simulink model "Model_3b_NH3_Flexible_clean"  (R2019a)
settings: Solver=FixedStepAuto  StartTime=0.0  StopTime=8760  FixedStep=1  RelTol=1e-3
libraries: simulink x8
settings Model: Creator=senja  LastModifiedBy=senja

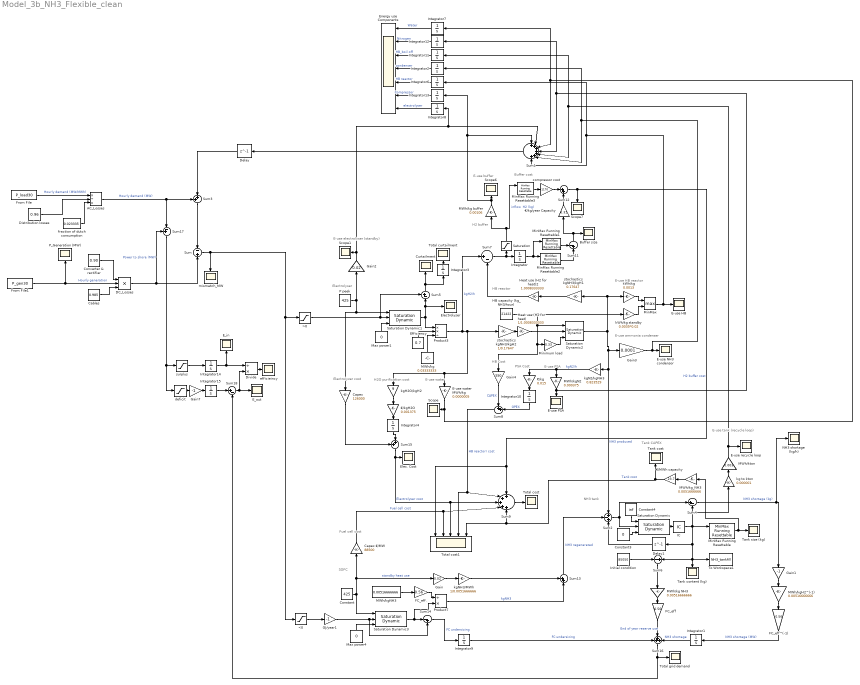
== system Model_3b_NH3_Flexible_clean ==
  note: PSA Cost
  note: H2O purification cost
  note: E-use buffer
  note: Buffer cost
  note: E-use HB reactor
  note: E-use PSA
  note: HB Cost
  note: Tank CAPEX
  note: E-use tank (recycle loop)
  note: E-use ammonia condenser
  note: NH3 tank
  note: HB reactor
  note: E-use electrolyser (standby)
  note: E-use water
  note: Fuel cell cost
  note: SOFC
  note: Electrolyser
  note: Electrolyzer cost
  note: H2 buffer
  " Heat use (H2 for heat)" : Gain  Gain=1/1.0008333333
  " Heat use (H2 for heat)2" : Gain  Gain=1.0008333333
  <0 : Saturate  UpperLimit=inf  LowerLimit=0
  >0 : Saturate  UpperLimit=inf  LowerLimit=0
  AC_Losses : Product  Inputs=*/*
  Buffer size : Scope
  Cables : Constant  Value=0.985
  Capex : Gain  Gain=126000
  Capex €/MW : Gain  Gain=88500
  Constant : Constant  Value=425
  Constant3 : Constant  Value=0
  Constant4 : Constant  Value=inf
  Converter & rectifier : Constant  Value=0.90
  Curtailment : Scope
  DC_Losses : Product  Inputs=3
  Delay : Delay  DelayLength=1  InitialCondition=0
  Delay1 : Delay  DelayLength=1
  Distribution losses : Constant  Value=0.96
  Divide : Product  Inputs=/*
  E-use HB : Scope
  E-use NH3 condensor : Scope
  E-use PSA : Scope
  E-use recycle loop : Scope
  E-use water MWh/kg : Gain  Gain=0.0000005
  E_in : Scope
  E_out : Scope
  Efficiency : Constant  Value=0.7
  Elec. Cost : Scope
  Electrolyser : Scope
  Energy use Components : Scope  NumInputPorts=7
  "FC_eff " : Gain  Gain=0.56
  FC_eff. : Gain  Gain=0.56
  FC_eff^(-1) : Gain  Gain=0.56
  From File : FromFile  FileName=P_load30  SampleTime=0
  From File1 : FromFile  FileName=P_gen30  SampleTime=0
  GJ/year1 : Gain  Gain=-1
  Gain : Gain  Gain=0.02
  Gain1 : Gain  Gain=-1
  Gain2 : Gain  Gain=0.02
  Gain3 : Gain  Gain=0.0001
  Gain4 : Gain  Gain=550
  Gain7 : Gain  Gain=-1
  HB capacity (kg_NH3/hour) : Constant  Value=21422
  IC : InitialCondition  Value=85050
  Initial condition : Constant  Value=85050
  Integrator{,1..4,6..15} (15 alike) : Integrator
  MWh/kg : Constant  Value=0.03333333
  MWh/kg buffer : Gain  Gain=0.00106
  MWh/kg NH3 : Gain  Gain=0.00516666666
  MWh/kgH2^(-1) : Gain  Gain=0.00516666666
  MWh/kgN2 : Gain  Gain=0.000375
  MWh/kgNH3 : Constant  Value=0.00516666666
  MWh/kg_NH3 : Gain  Gain=0.0051666666
  MWh/kton : Gain  Gain=0.003
  Max power1 : Constant  Value=0
  Max power4 : Constant  Value=0
  MinMax : MinMax  Function=max  Inputs=2
  MinMax Running Resettable : simulink/Math Operations/MinMax Running Resettable  Function=max  vinit=0.0
  MinMax Running Resettable1 : simulink/Math Operations/MinMax Running Resettable  Function=min  vinit=0.0
  MinMax Running Resettable2 : simulink/Math Operations/MinMax Running Resettable  Function=max  vinit=0.0
  MinMax Running Resettable3 : simulink/Math Operations/MinMax Running Resettable  Function=max  vinit=0.0
  Minimum load : Gain  Gain=0.33
  NH3 shortage (kg/h) : Scope
  P peek : Constant  Value=425
  P_Generation (MW) : Scope
  Product3 : Product  Inputs=**/
  Product7 : Product  Inputs=/*
  Saturation : Saturate  UpperLimit=inf  LowerLimit=0
  Saturation Dynamic{,1..3} (4 alike) : simulink/Discontinuities/Saturation Dynamic  OutMin=[]  OutMax=[]  OutDataTypeStr=Inherit: Same as second input  OutDataType=fixdt(1, 16)  OutScaling=2^-10  DoSatur=off
  Scope{,1,6..7} (4 alike) : Scope
  Sum : Sum  Inputs=-|+
  Sum1 : Sum  Inputs=+++++++
  Sum11 : Sum  Inputs=-+|
  Sum12 : Sum  Inputs=|++
  Sum{3,8,13,15} (4 alike) : Sum  Inputs=++|
  Sum14 : Sum  Inputs=|-+
  Sum16 : Sum  Inputs=+++
  Sum17 : Sum  Inputs=+-|
  Sum18 : Sum  Inputs=|+-
  Sum2 : Sum  Inputs=+-+
  Sum4 : Sum  Inputs=|+-
  Sum5 : Sum  Inputs=+-|
  Sum6 : Sum  Inputs=-|+
  Sum7 : Sum  Inputs=|+-
  Sum9 : Sum  Inputs=+++++
  Tank content (kg) : Scope
  Tank cost : Scope
  Tank size (kg) : Scope
  To Workspace1 : ToWorkspace  VariableName=NH3_tankfill  SampleTime=-1
  Total cost : Scope
  Total cost1 : Scope  NumInputPorts=5
  Total curtailment : Scope
  Total grid demand : Scope
  compressor cost : Gain  Gain=1170
  deficit : Saturate  UpperLimit=0  LowerLimit=-inf
  efficieincy : Scope
  fraction of dutch consumption : Constant  Value=0.023335
  kWh/kg : Gain  Gain=0.0013
  kWh/kg standby : Gain  Gain=0.0035*0.02
  kg to kton : Gain  Gain=0.000001
  kgH2O/kgH2 : Gain  Gain=9
  kgN2/kgNH3 : Gain  Gain=0.823529
  kgNH3/MWh : Gain  Gain=1/0.0051666666
  mismatch_MW : Scope
  stochastics kgNH3/kgH1 : Gain  Gain=0.17647
  stochastics kgNH3/kgH2 : Gain  Gain=1/0.17647
  surplus : Saturate  UpperLimit=inf  LowerLimit=0
  €/MWh capacity : Gain  Gain=23.7
  €/kg : Gain  Gain=0.015
  €/kg/year Capacity : Gain  Gain=0.31
  €/kgH2O : Gain  Gain=0.001375
  wires:
  From File/1 -> AC_Losses/1  "Hourly demand (MW/MWh)"
  Efficiency/1 -> Product3/2
  fraction of dutch consumption/1 -> AC_Losses/3
  Distribution losses/1 -> AC_Losses/2
  Cables/1 -> DC_Losses/3
  Converter & rectifier/1 -> DC_Losses/1
  DC_Losses/1 -> Sum/2, Sum17/1  "Power to shore (MW)"
  >0/1 -> Sum5/1, Saturation Dynamic1/2
  <0/1 -> GJ/year1/1
  AC_Losses/1 -> Sum3/1, Sum17/2  "Hourly demand (MW)"
  From File1/1 -> P_Generation (MW)/1, DC_Losses/2  "Hourly generation"
  Max power1/1 -> Saturation Dynamic1/3
  Saturation Dynamic1/1 -> Electrolyser/1, Sum5/2, Product3/1
  Capex/1 -> Sum15/1
  Sum15/1 -> Elec. Cost/1, Total cost1/3, Sum9/3  "Electrolyser cost"
  €/kgH2O/1 -> Integrator4/1
  P peek/1 -> Saturation Dynamic1/1, Capex/1, Gain2/1
  GJ/year1/1 -> Saturation Dynamic3/2, Sum14/2
  Product3/1 -> stochastics kgNH3/kgH2/1, E-use water MWh/kg/1, kgH2O/kgH2/1, Sum7/1  "kgH2/h"
  Sum/1 -> <0/1, >0/1, mismatch_MW/1
  Sum9/1 -> Total cost/1
  Constant/1 -> Saturation Dynamic3/1, Capex €/MW/1, Gain/1  "standby heat use"
  Max power4/1 -> Saturation Dynamic3/3
  Saturation Dynamic3/1 -> Sum14/1, Product7/2
  MWh/kgNH3/1 -> FC_eff./1
  Integrator3/1 -> Total curtailment/1
  kgH2O/kgH2/1 -> €/kgH2O/1
  Integrator4/1 -> Sum15/2
  MWh/kg/1 -> Product3/3
  Capex €/MW/1 -> Total cost1/2, Sum9/4  "Fuel cell cost"
  FC_eff./1 -> Product7/1
  Sum5/1 -> Curtailment/1, Integrator3/1
  E-use water MWh/kg/1 -> Sum1/3, Integrator7/1, Scope/1
  Gain2/1 -> Integrator8/1, Sum1/2, Scope1/1
  Sum3/1 -> Sum/1
  Sum1/1 -> Delay/1
  Delay/1 -> Sum3/2
  Integrator2/1 -> Energy use Components/4  "condenser"
  Integrator6/1 -> Energy use Components/5  "HB reactor"
  Integrator7/1 -> Energy use Components/1  "Water"
  Integrator8/1 -> Energy use Components/7  "electrolyser"
  Product7/1 -> Sum13/2  "kgNH3"
  Sum7/1 -> Integrator/1, Saturation/1
  Integrator/1 -> MinMax Running Resettable1/1, MinMax Running Resettable2/1
  stochastics kgNH3/kgH2/1 -> " Heat use (H2 for heat)"/1
  HB capacity (kg_NH3/hour)/1 -> Saturation Dynamic2/1, Gain4/1, Minimum load/1, kWh/kg standby/1
  Sum2/1 -> Sum4/1, Saturation Dynamic/2
  Delay1/1 -> Sum2/3
  Constant3/1 -> Saturation Dynamic/3
  Sum4/1 -> NH3 shortage (kg/h)/1, Gain1/1  "NH3 shortage (kg)"
  MWh/kgH2^(-1)/1 -> FC_eff^(-1)/1
  FC_eff^(-1)/1 -> Integrator1/1  "NH3 shortage (MW)"
  Saturation Dynamic/1 -> IC/1
  IC/1 -> Sum4/2, kg to kton/1, Tank content (kg)/1, Sum6/2, To Workspace1/1, Delay1/1, MinMax Running Resettable/1
  Initial condition/1 -> Sum6/1
  Sum14/1 -> Integrator9/1  "FC undersizing"
  MWh/kg NH3/1 -> "FC_eff "/1
  "FC_eff "/1 -> Sum16/2  "End of year reserve use"
  Sum6/1 -> MWh/kg NH3/1
  Gain1/1 -> MWh/kgH2^(-1)/1
  Integrator9/1 -> Sum16/1  "FC undersizing"
  Constant4/1 -> Saturation Dynamic/1
  MinMax Running Resettable/1 -> Tank size (kg)/1, MWh/kg_NH3/1
  Gain3/1 -> Sum1/6, Integrator2/1, E-use NH3 condensor/1
  MWh/kton/1 -> Sum1/5, Integrator11/1, E-use recycle loop/1
  kg to kton/1 -> MWh/kton/1
  MWh/kg_NH3/1 -> €/MWh capacity/1
  €/MWh capacity/1 -> Total cost1/5, Sum9/5, Tank cost/1  "Tank cost"
  Gain4/1 -> Sum8/1  "CAPEX"
  kgN2/kgNH3/1 -> MWh/kgN2/1, €/kg/1  "kgN2/h"
  €/kg/1 -> Integrator10/1
  Sum8/1 -> Total cost1/4, Sum9/2  "HB reactorr cost"
  Integrator10/1 -> Sum8/2  "OPEX"
  kWh/kg/1 -> MinMax/1
  Integrator12/1 -> Energy use Components/2  "Nitrogen"
  Integrator11/1 -> Energy use Components/3  "HB_boil off"
  MWh/kgN2/1 -> Sum1/4, Integrator12/1, E-use PSA/1
  MinMax Running Resettable1/1 -> Sum11/1
  MinMax Running Resettable2/1 -> Sum11/2
  Sum11/1 -> Buffer size/1, €/kg/year Capacity/1
  €/kg/year Capacity/1 -> Sum12/2
  MWh/kg buffer/1 -> Sum1/1, Integrator13/1, Scope6/1
  Saturation/1 -> MinMax Running Resettable3/1, MWh/kg buffer/1  "inflow  H2 (kg)"
  MinMax Running Resettable3/1 -> compressor cost/1
  compressor cost/1 -> Sum12/1
  Sum12/1 -> Scope7/1, Total cost1/1, Sum9/1  "H2 buffer cost"
  Integrator13/1 -> Energy use Components/6  "Compressor"
  Sum13/1 -> Sum2/2  "NH3 regenerated"
  Gain/1 -> kgNH3/MWh/1
  kgNH3/MWh/1 -> Sum13/1
  kWh/kg standby/1 -> MinMax/2
  MinMax/1 -> Sum1/7, Integrator6/1, E-use HB/1
  " Heat use (H2 for heat)"/1 -> Saturation Dynamic2/2
  Minimum load/1 -> Saturation Dynamic2/3
  Saturation Dynamic2/1 -> stochastics kgNH3/kgH1/1, kWh/kg/1, Gain3/1, Sum2/1, kgN2/kgNH3/1  "NH3 produced"
  stochastics kgNH3/kgH1/1 -> " Heat use (H2 for heat)2"/1
  " Heat use (H2 for heat)2"/1 -> Sum7/2
  Sum16/1 -> Sum18/2, Total grid demand/1
  Integrator14/1 -> E_in/1, Divide/1
  Integrator15/1 -> Sum18/1
  Sum18/1 -> Divide/2, E_out/1
  Gain7/1 -> Integrator15/1
  deficit/1 -> Gain7/1
  Sum17/1 -> surplus/1, deficit/1
  surplus/1 -> Integrator14/1
  Divide/1 -> efficieincy/1
  Integrator1/1 -> Sum16/3  "NH3 shortage"
